simulink subsystem "airframe_weight"  (R2023b)
settings: Solver=VariableStepAuto  StartTime=0.0  StopTime=10.0  RelTol=1e-3
undefined symbols (not defined in the file): mass
libraries: sharedtransform x1
settings Model: Creator=Victor  LastModifiedBy=Victor

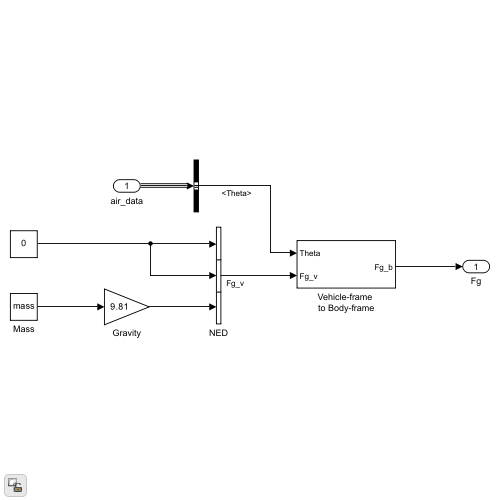
[thumbnail: Simulink's stored preview of the top-level diagram]
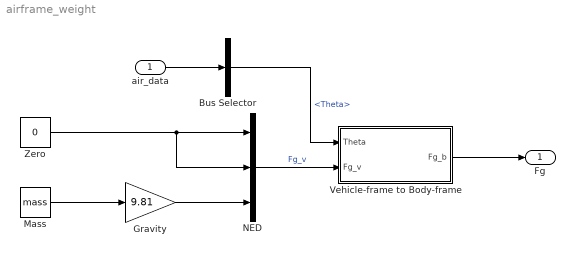
== system airframe_weight ==
  air_data : Inport
  Bus Selector : BusSelector  OutputSignals=state.Theta
  Gravity : Gain  Gain=9.81
  Mass : Constant  Value=mass
  NED : Concatenate  NumInputs=3
  Vehicle-frame to Body-frame : Subsystem
  Zero : Constant  Value=0  OutDataTypeStr=Inherit: Inherit via back propagation
  Fg : Outport
  wires:
  Bus Selector/1 -> Vehicle-frame to Body-frame/1(Theta)  "<Theta>"
  air_data/1 -> Bus Selector/1
  Vehicle-frame to Body-frame/1(Fg_b) -> Fg/1
  NED/1 -> Vehicle-frame to Body-frame/2(Fg_v)  "Fg_v"
  Zero/1 -> NED/1, NED/2
  Gravity/1 -> NED/3
  Mass/1 -> Gravity/1

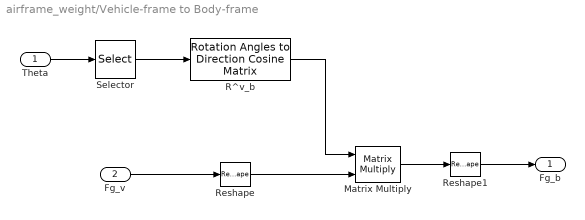
== system airframe_weight/Vehicle-frame to Body-frame ==
  Theta : Inport
  Fg_v : Inport  Port=2
  Matrix Multiply : Product  Multiplication=Matrix(*)
  R^v_b : sharedtransform/Rotation Angles to Direction Cosine Matrix  rotationOrder=ZYX  aMode=aMode
  Reshape : Reshape  OutputDimensionality=Column vector (2-D)
  Reshape1 : Reshape
  Selector : Selector  InputPortWidth=3  IndexOptions=Index vector (dialog)  Indices=[3 2 1]  OutputSizes=1
  Fg_b : Outport
  wires:
  Matrix Multiply/1 -> Reshape1/1
  Theta/1 -> Selector/1
  Selector/1 -> R^v_b/1
  R^v_b/1 -> Matrix Multiply/1
  Fg_v/1 -> Reshape/1
  Reshape/1 -> Matrix Multiply/2
  Reshape1/1 -> Fg_b/1
